simulink model "single_thruster"  (R2022b)
settings: Solver=VariableStepAuto  StartTime=0.0  StopTime=21  RelTol=1e-3
libraries: simulink x1, MarineRoboticsLib x1
settings Model: Creator=dnad  LastModifiedBy=dnad

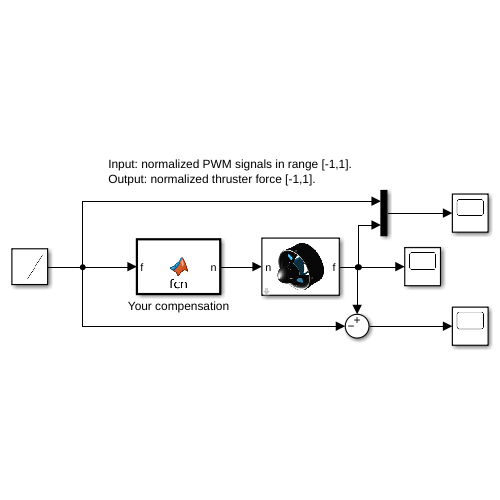
[thumbnail: Simulink's stored preview of the top-level diagram]
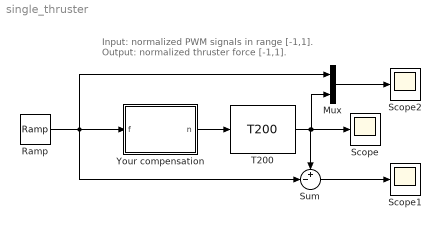
== system single_thruster ==
  note: Input: normalized PWM signals in range [-1,1].
      | Output: normalized thruster force [-1,1].
  Mux : Mux  Inputs=2
  Ramp : simulink/Sources/Ramp  slope=0.1  start=1  InitialOutput=-0.7
  Scope : Scope
  Scope1 : Scope
  Scope2 : Scope
  Sum : Sum  Inputs=+-|
  T200 : MarineRoboticsLib/T200  Keff=1  Tm=0
  Your compensation : MATLAB Function  TreatAsAtomicUnit=on
  wires:
  Ramp/1 -> Your compensation/1(f), Sum/2, Mux/1
  Mux/1 -> Scope2/1
  Sum/1 -> Scope1/1
  Your compensation/1(n) -> T200/1
  T200/1 -> Mux/2, Scope/1, Sum/1

== matlab function single_thruster/Your compensation ==
  data: f input; n output
function n = fcn(f)

n = f;

end
